simulink model "receive_nad_r2017b"  (R2017b)
settings: Solver=VariableStepAuto  StartTime=0.0  StopTime=10.0  RelTol=1e-3
model workspace (MAT data in the model file):
  ED247Configuration(1).name = 'Signal00'
  ED247Configuration(1).direction = 'IN'
  ED247Configuration(1).type = 'uint8'
  ED247Configuration(1).dimensions = 1
  ED247Configuration(1).width = 1
  ED247Configuration(1).size = 1
  ED247Configuration(1).sample_time = 0.00999999977648
  ED247Configuration(1).validity_duration = 0
  ED247Configuration(1).signal_type = 'NAD'
  ED247Configuration(1).sample_size = 1
  ED247Configuration(2).name = 'Signal01'
  ED247Configuration(2).direction = 'IN'
  ED247Configuration(2).type = 'uint8'
  ED247Configuration(2).dimensions = 1
  ED247Configuration(2).width = 1
  ED247Configuration(2).size = 1
  ED247Configuration(2).sample_time = 0.00999999977648
  ED247Configuration(2).validity_duration = 0
  ED247Configuration(2).signal_type = 'NAD'
  ED247Configuration(2).sample_size = 1
  ED247Configuration(3).name = 'Signal11'
  ED247Configuration(3).direction = 'IN'
  ED247Configuration(3).type = 'single'
  ED247Configuration(3).dimensions = 2
  ED247Configuration(3).width = 4
  ED247Configuration(3).size = [2 2]
  ED247Configuration(3).sample_time = 0.00999999977648
  ED247Configuration(3).validity_duration = 0
  ED247Configuration(3).signal_type = 'NAD'
  ED247Configuration(3).sample_size = 16
libraries: lib_ed247 x2
settings Model: Creator=odufour  LastModifiedBy=odufour
settings DataIOCC: ExternalInput=ds  ReturnWorkspaceOutputs=on
settings DebuggingCC: InheritedTsInSrcMsg=none
settings SFSimCC: SimUseLocalCustomCode=on
settings RTWCC: RTWUseLocalCustomCode=on

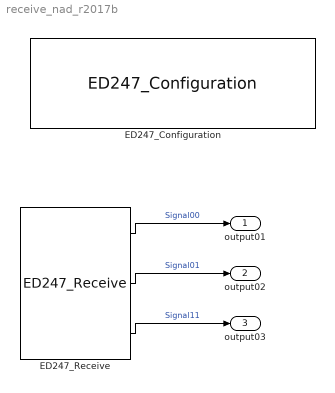
== system receive_nad_r2017b ==
  ED247_Configuration : lib_ed247/ED247_Configuration  configurationFilename='ecic_func_exchange_nad_uc_tester.xml'  enableLog=off  logFilename=''
      settings: SourceProductName=Airbus ED247
  ED247_Receive : lib_ed247/ED247_Receive  enable_refresh=on  refresh_factor=1  sample_time=-1  show_port_labels=on
      settings: SourceProductName=Airbus ED247
  output01 : Outport  OutDataTypeStr=uint8
  output02 : Outport  Port=2  OutDataTypeStr=uint8
  output03 : Outport  Port=3  OutDataTypeStr=single  PortDimensions=[2,2]
  wires:
  ED247_Receive/1 -> output01/1  "Signal00"
  ED247_Receive/2 -> output02/1  "Signal01"
  ED247_Receive/3 -> output03/1  "Signal11"
